simulink model "Michaels_CVModel_fast8"  (R2020a)
settings: Solver=ode23  StartTime=0.0  StopTime=30  RelTol=1e-2  EnableMultiTasking=on
model workspace (MAT data in the model file):
  Eao = 1.88
  Eesla = 0.58
  Eeslvf = 5.2
  Eesra = 0.63
  Eesrvf = 1.75
  Emaxspt = 48.75
  Epa = 0.15
  Epu = 0.04
  Esa = 0.37
  Esv = 0.013
  Evc = 0.03
  GpLV = 0
  GpRR = 11
  GpRV = 0
  GpRsa = 0
  GpV0 = 0
  GsLV = 0.007
  GsRR = 11
  GsRV = 0.022
  GsRsa = -0.05
  GsV0 = 31
  Ka = 4.4
  Lao = 0.0022
  Lav = 0.000354
  Lmt = 7.697e-05
  Lpa = 7.697e-05
  Lpv = 0.0001043
  Ltc = 8.009e-05
  P0la = 0.5
  P0lvf = 0.98
  P0pcd = 0.5
  P0ra = 0.5
  P0rvf = 0.91
  P0spt = 0.46
  PV : AO (value not decoded)
  PVao = [327.9; 100.9]
  Rao = 0.28
  Rav = 0.02
  Rla2pu = 0.5
  Rmt = 0.01
  Rpa = 0.12
  Rpa_Vals = 0.12
  Rpu = 0.006
  Rpv = 0.02
  Rra = 0.012
  Rsa = 0.74
  Rsv = 0.12
  Rtc = 0.01
  Tc = 1
  Tsys0 = 0.6
  V0la = 30
  V0lvf = 45
  V0pcd = 200
  V0ra = 25
  V0rvf = 50
  V0spt = 10
  Vdla = 15
  Vdlvf = 16
  Vdra = 15
  Vdrvf = 40
  Vdspt = 10
  Vlv0 = 100
  Vperi = 51
  Vrv0 = 105
  Vuao = 260.8
  Vupa = 91
  Vupu = 132
  Vusa = 287.4
  Vusv = 1976.1
  Vuvc = 136.17
  amin = -2
  artBrLVcontConti = []
  artBrLVcontDigi = [0 0 0 0 0 0 0 0 0 0 0 0 ... (240 elements, 1x240)]
  artBrRRConti = []
  artBrRRDigi = [0 0 0 0 0 0 0 0 0 0 1.57142857143 3.14285714286 ... (240 elements, 1x240)]
  artBrRVcontConti = []
  artBrRVcontDigi = [0 0 0 0 0 0 0 0 0 0 0 0 ... (240 elements, 1x240)]
  artBrRsaConti = []
  artBrRsaDigi = [0 0 0 0 0 0 0 0 0 0 0 0 ... (480 elements, 1x480)]
  artBrV0Conti = []
  artBrV0Digi = [0 0 0 0 0 0 0 0 0 0 0 0 ... (640 elements, 1x640)]
  atriumA = 1
  baroSampFreq = 16
  cP0la = 0.5
  cP0lvf = 0.98
  cP0ra = 0.5
  cP0rvf = 0.91
  cT = 1
  cVtotal = 5400
  clambdala = 0.13
  clambdalvf = 0.028
  clambdara = 0.13
  clambdarvf = 0.028
  deac = 0.0004
  ksys = 0.075
  lambdala = 0.065
  lambdalvf = 0.042
  lambdapcd = 0.005
  lambdara = 0.065
  lambdarvf = 0.028
  lambdaspt = 0.4
  pThor = 0
  params : object (value not decoded)
  sampleTime = 0.005
  svcPressureChange_MCS = 0
  svrMult = 1
  tStepOn = 1000000000
  t_baroOn = 1000000
  t_testBed_start = 1000000
  venk1 = 0.5
  venk2 = 0.5
symbols that are objects in the model workspace (value not decoded): PV
undefined symbols (not defined in the file): dfilt
libraries: simulink x85, fl_lib x39, nesl_utility x24, cstblocks x9, dspstat3 x9, dspobslib x5, SimscapeFluids_lib x5, sh_lib x1
(part 3 of 5)

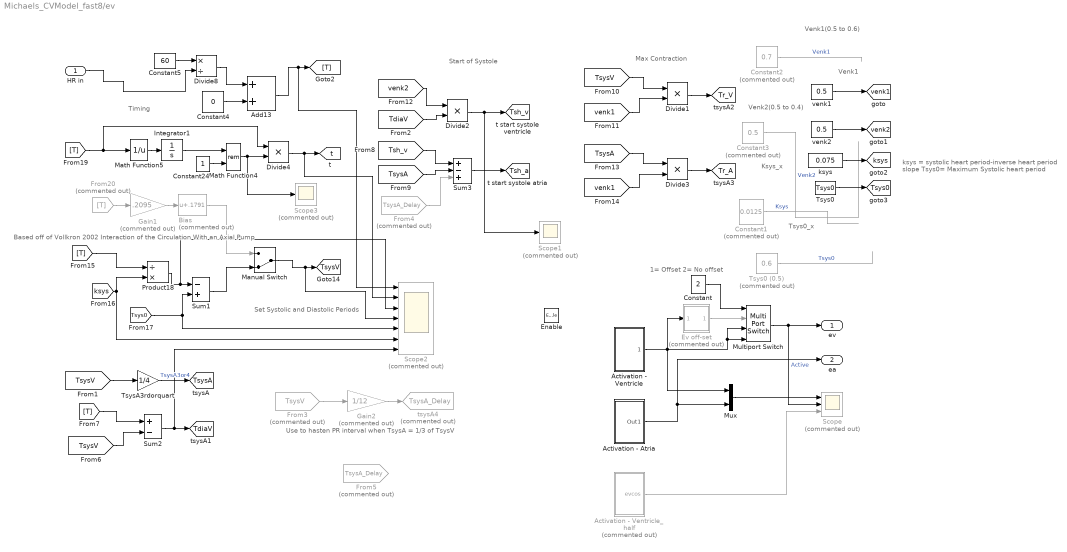
== system Michaels_CVModel_fast8/ev ==
  note: 1= Offset
      | 2= No offset
  note: ksys = systolic heart period-inverse heart period slope
      |
      | Tsys0= Maximum Systolic heart period
  note: Venk1(0.5 to 0.6)
  note: Ksys_x
  note: Timing
  note: Set Systolic and Diastolic Periods
  note: Start of Systole
  note: Max Contraction
  note: Venk1
  note: Based off of Vollkron 2002 Interaction of the Circulation With an Axial Pump
  note: Tsys0_x
  note: Venk2(0.5 to 0.4)
  note: Use to hasten PR interval when TsysA = 1/3 of TsysV
  HR in : Inport
  Enable : EnablePort
  Activation - Atria : Subsystem
  Activation - Ventricle : Subsystem
  Activation - Ventricle_half : Subsystem  Commented=on
  Add13 : Sum
  Bias : Bias  Commented=on  Bias=.1791
  Constant : Constant  Value=2
  Constant1 : Constant  Description=SettingsEV  Commented=on  Value=0.0125
  Constant2 : Constant  Description=SettingsEV  Commented=on  Value=0.7
  Constant24 : Constant
  Constant3 : Constant  Description=SettingsEV  Commented=on  Value=0.5
  Constant4 : Constant  Value=0
  Constant5 : Constant  Value=60
  Divide{1..4} (4 alike) : Product  Inputs=**
  Divide8 : Product  Inputs=*/
  Ev off-set : Subsystem  Commented=on
  From20 : From  Commented=on  GotoTag=T
      settings: CloseFcn=tagdialog Close
  From3 : From  Commented=on  GotoTag=TsysV  TagVisibility=global
      settings: CloseFcn=tagdialog Close
  From4 : From  Commented=on  GotoTag=TsysA_Delay
      settings: CloseFcn=tagdialog Close
  From5 : From  Commented=on  GotoTag=TsysA_Delay  TagVisibility=global
      settings: CloseFcn=tagdialog Close
  Gain1 : Gain  Commented=on  Gain=.2095
  Gain2 : Gain  Commented=on  Gain=1/12
  Integrator1 : Integrator
  Manual Switch : ManualSwitch  CurrentSetting=0
  Math Function4 : Math  Operator=rem  SignedPower=on  SaturateOnIntegerOverflow=on
  Math Function5 : Math  Operator=reciprocal  SignedPower=on  SaturateOnIntegerOverflow=on
  Multiport Switch : MultiPortSwitch
  Mux : Mux  Inputs=2
  Product18 : Product  Inputs=/*  InputSameDT=on  RndMeth=Zero  SaturateOnIntegerOverflow=on  OutDataTypeStr=Inherit: Same as first input
  Scope : Scope  Commented=on  NumInputPorts=3
  Scope1 : Scope  Commented=on
  Scope2 : Scope  Commented=on  NumInputPorts=7
  Scope3 : Scope  Commented=on
  Sum1 : Sum  Inputs=-+  InputSameDT=on  SaturateOnIntegerOverflow=on  OutDataTypeStr=Inherit: Same as first input
  Sum2 : Sum  Inputs=+-  InputSameDT=on  SaturateOnIntegerOverflow=on  OutDataTypeStr=Inherit: Same as first input
  Sum3 : Sum  Inputs=+-+  InputSameDT=on  SaturateOnIntegerOverflow=on  OutDataTypeStr=Inherit: Same as first input
  Tsys0 : Constant  Value=Tsys0
  Tsys0 (0.5) : Constant  Description=SettingsEV  Commented=on  Value=0.6
  TsysA3rdorquart : Gain  Gain=1/4
  ksys : Constant  Value=0.075
  tsysA4 : Goto  Commented=on  GotoTag=TsysA_Delay  TagVisibility=global
  venk1 : Constant  Value=0.5
  venk2 : Constant  Value=0.5
  ev : Outport  InitialOutput=0
  ea : Outport  Port=2  InitialOutput=0
  tag scope: TdiaV=global, Tr_A=global, Tr_V=global, Tsh_a=global, Tsh_v=global, Tsys0=global, TsysA=global, TsysV=global, ksys=global, t=global, venk1=global, venk2=global
  wires:
  [Tsys0] -> Sum1/2, Scope2/5
  Product18/1 -> Scope2/3, Sum1/1
  [ksys] -> Product18/2, Scope2/6
  Constant24/1 -> Math Function4/2
  Math Function5/1 -> Integrator1/1
  Integrator1/1 -> Math Function4/1
  [T] -> Math Function5/1, Divide4/1
  Math Function4/1 -> Scope3/1, Divide4/2
  Constant5/1 -> Divide8/1
  [TsysV] -> TsysA3rdorquart/1
  TsysA3rdorquart/1 -> [TsysA]  "TsysA3or4"
  [T] -> Sum2/1
  [TsysV] -> Sum2/2
  Sum2/1 -> Scope2/7, [TdiaV]
  [TdiaV] -> Divide2/2
  Divide2/1 -> [Tsh_v], Scope1/1
  [Tsh_v] -> Sum3/1
  [TsysA] -> Sum3/2
  Sum3/1 -> [Tsh_a]
  [TsysV] -> Divide1/1
  [venk1] -> Divide1/2
  [venk2] -> Divide2/1
  Divide1/1 -> [Tr_V]
  [TsysA] -> Divide3/1
  [venk1] -> Divide3/2
  Divide3/1 -> [Tr_A]
  [T] -> Product18/1
  Divide4/1 -> Scope2/2, [t]
  Sum1/1 -> Manual Switch/2
  Manual Switch/1 -> Scope2/4, [TsysV]
  From20/1 -> Gain1/1
  Gain1/1 -> Bias/1
  Bias/1 -> Manual Switch/1
  Mux/1 -> Scope/1
  Activation - Atria/1(Out1) -> ea/1, Mux/2
  HR in/1 -> Divide8/2
  Divide8/1 -> Add13/1
  Add13/1 -> Scope2/1, [T]
  Constant1/1 -> ?  "Ksys"
  Tsys0 (0.5)/1 -> ?  "Tsys0"
  Constant2/1 -> ?  "Venk1"
  Constant3/1 -> ?  "Venk2"
  Activation - Ventricle/1(1) -> Multiport Switch/4, Multiport Switch/3, Mux/1, Ev off-set/1(Inport)
  Activation - Ventricle_half/1(evcos) -> Scope/3
  Constant/1 -> Multiport Switch/1
  Ev off-set/1(" ") -> Multiport Switch/2
  Multiport Switch/1 -> Scope/2, ev/1  "Active"
  Constant4/1 -> Add13/2
  Gain2/1 -> tsysA4/1
  From3/1 -> Gain2/1
  From4/1 -> Sum3/3
  venk1/1 -> [venk1]
  venk2/1 -> [venk2]
  ksys/1 -> [ksys]
  Tsys0/1 -> [Tsys0]

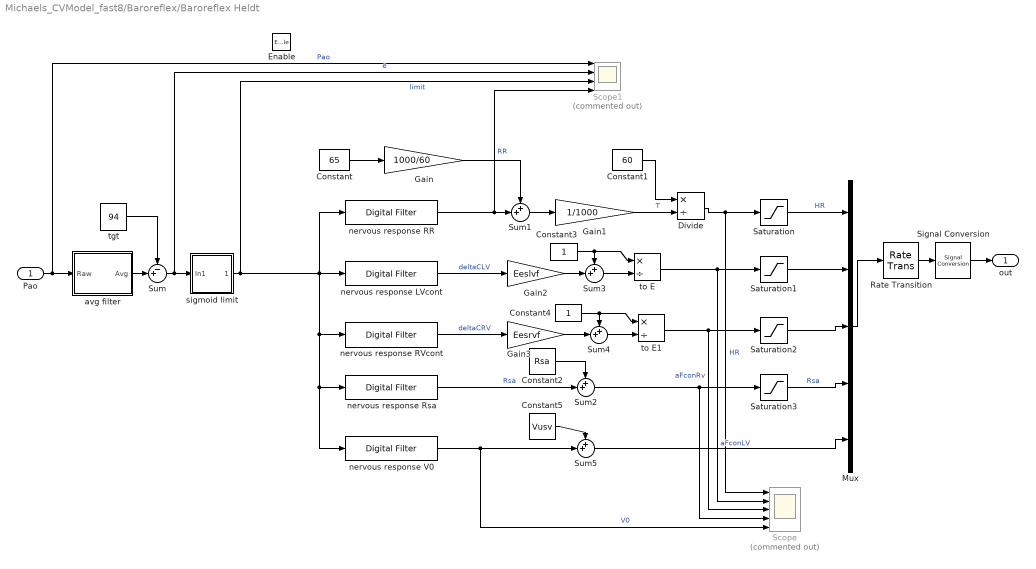
== system Michaels_CVModel_fast8/Baroreflex/Baroreflex Heldt ==
  Pao : Inport
  Enable : EnablePort
  Constant : Constant  Value=65
  Constant1 : Constant  Value=60
  Constant2 : Constant  Value=Rsa
  Constant3 : Constant
  Constant4 : Constant
  Constant5 : Constant  Value=Vusv
  Divide : Product  Inputs=*/
  Gain : Gain  Gain=1000/60
  Gain1 : Gain  Gain=1/1000
  Gain2 : Gain  Gain=Eeslvf
  Gain3 : Gain  Gain=Eesrvf
  Mux : Mux  Inputs=5
  Rate Transition : RateTransition  InitialCondition=[60,1,1,0.74,2000]
  Saturation : Saturate  UpperLimit=200  LowerLimit=30
  Saturation1 : Saturate  UpperLimit=10  LowerLimit=0.01
  Saturation2 : Saturate  UpperLimit=10  LowerLimit=0.01
  Saturation3 : Saturate  UpperLimit=inf  LowerLimit=0.001
  Scope : Scope  Commented=on  NumInputPorts=5
  Scope1 : Scope  Commented=on  NumInputPorts=4
  Signal Conversion : SignalConversion  OverrideOpt=off
  Sum : Sum  Inputs=-+|
  Sum{1..5} (5 alike) : Sum  Inputs=++|
  avg filter : Subsystem
  nervous response LVcont : dspobslib/Digital Filter  TypePopup=FIR (all zeros)  IIRFiltStruct=Direct form I  AllPoleFiltStruct=Direct form  FIRFiltStruct=Direct form  CoeffSource=Specify via dialog  NumCoeffs=artBrLVcontDigi  DenCoeffs=[1]  BiQuadCoeffs=[1 0.3 0.4 1 0.1 0.2]  LatticeCoeffs=[0.2 0.4]  denIgnore=on  FiltPerSampPopup=One filter per frame  IC=0  ICnum=0  ICden=0  roundingMode=Floor  overflowMode=off  ScaleValues=1  scaleValueFracLength=14  stageInFracLength=15  stageOutFracLength=15  FilterSource=Specify via dialog  dfiltObjectName=dfilt.dffir([1 2 1])
      settings: SourceProductBaseCode=DS
  nervous response RR : dspobslib/Digital Filter  TypePopup=FIR (all zeros)  IIRFiltStruct=Direct form I  AllPoleFiltStruct=Direct form  FIRFiltStruct=Direct form  CoeffSource=Specify via dialog  NumCoeffs=artBrRRDigi  DenCoeffs=[1]  BiQuadCoeffs=[1 0.3 0.4 1 0.1 0.2]  LatticeCoeffs=[0.2 0.4]  denIgnore=on  FiltPerSampPopup=One filter per frame  IC=0  ICnum=0  ICden=0  roundingMode=Floor  overflowMode=off  ScaleValues=1  scaleValueFracLength=14  stageInFracLength=15  stageOutFracLength=15  FilterSource=Specify via dialog  dfiltObjectName=dfilt.dffir([1 2 1])  InputProcessing=Columns as channels (frame based)
      settings: SourceProductBaseCode=DS
  nervous response RVcont : dspobslib/Digital Filter  TypePopup=FIR (all zeros)  IIRFiltStruct=Direct form I  AllPoleFiltStruct=Direct form  FIRFiltStruct=Direct form  CoeffSource=Specify via dialog  NumCoeffs=artBrRVcontDigi  DenCoeffs=[1]  BiQuadCoeffs=[1 0.3 0.4 1 0.1 0.2]  LatticeCoeffs=[0.2 0.4]  denIgnore=on  FiltPerSampPopup=One filter per frame  IC=0  ICnum=0  ICden=0  roundingMode=Floor  overflowMode=off  ScaleValues=1  scaleValueFracLength=14  stageInFracLength=15  stageOutFracLength=15  FilterSource=Specify via dialog  dfiltObjectName=dfilt.dffir([1 2 1])
      settings: SourceProductBaseCode=DS
  nervous response Rsa : dspobslib/Digital Filter  TypePopup=FIR (all zeros)  IIRFiltStruct=Direct form I  AllPoleFiltStruct=Direct form  FIRFiltStruct=Direct form  CoeffSource=Specify via dialog  NumCoeffs=artBrRsaDigi  DenCoeffs=[1]  BiQuadCoeffs=[1 0.3 0.4 1 0.1 0.2]  LatticeCoeffs=[0.2 0.4]  denIgnore=on  FiltPerSampPopup=One filter per frame  IC=0  ICnum=0  ICden=0  roundingMode=Floor  overflowMode=off  ScaleValues=1  scaleValueFracLength=14  stageInFracLength=15  stageOutFracLength=15  FilterSource=Specify via dialog  dfiltObjectName=dfilt.dffir([1 2 1])
      settings: SourceProductBaseCode=DS
  nervous response V0 : dspobslib/Digital Filter  TypePopup=FIR (all zeros)  IIRFiltStruct=Direct form I  AllPoleFiltStruct=Direct form  FIRFiltStruct=Direct form  CoeffSource=Specify via dialog  NumCoeffs=artBrV0Digi  DenCoeffs=[1]  BiQuadCoeffs=[1 0.3 0.4 1 0.1 0.2]  LatticeCoeffs=[0.2 0.4]  denIgnore=on  FiltPerSampPopup=One filter per frame  IC=0  ICnum=0  ICden=0  roundingMode=Floor  overflowMode=off  ScaleValues=1  scaleValueFracLength=14  stageInFracLength=15  stageOutFracLength=15  FilterSource=Specify via dialog  dfiltObjectName=dfilt.dffir([1 2 1])
      settings: SourceProductBaseCode=DS
  sigmoid limit : Subsystem
  tgt : Constant  Value=94
  to E : Product  Inputs=*/
  to E1 : Product  Inputs=*/
  out : Outport  InitialOutput=[60,1,1,0.74,2000]
  wires:
  Pao/1 -> avg filter/1(Raw), Scope1/1  "Pao"
  tgt/1 -> Sum/1
  avg filter/1(Avg) -> Sum/2
  Sum/1 -> Scope1/2, sigmoid limit/1(In1)  "e"
  nervous response RR/1 -> Sum1/2, Scope1/4  "RR"
  nervous response LVcont/1 -> Gain2/1  "deltaCLV"
  nervous response Rsa/1 -> Sum2/2  "Rsa"
  nervous response V0/1 -> Scope/5, Sum5/2  "V0"
  Constant/1 -> Gain/1
  Gain/1 -> Sum1/1
  Sum1/1 -> Gain1/1
  Divide/1 -> Saturation/1, Scope/1  "HR"
  Saturation/1 -> Mux/1  "HR"
  Constant1/1 -> Divide/1
  Gain1/1 -> Divide/2  "T"
  sigmoid limit/1(Out1) -> Scope1/3, nervous response RR/1, nervous response LVcont/1, nervous response RVcont/1, nervous response Rsa/1, nervous response V0/1  "limit"
  Constant2/1 -> Sum2/1
  Sum2/1 -> Scope/4, Saturation3/1
  Constant3/1 -> Sum3/1, to E/1
  Sum3/1 -> to E/2
  Gain2/1 -> Sum3/2
  to E/1 -> Scope/2, Saturation1/1  "aFconLV"
  Constant4/1 -> Sum4/1, to E1/1
  Sum4/1 -> to E1/2
  Gain3/1 -> Sum4/2
  nervous response RVcont/1 -> Gain3/1  "deltaCRV"
  to E1/1 -> Scope/3, Saturation2/1  "aFconRv"
  Saturation1/1 -> Mux/2
  Saturation2/1 -> Mux/3
  Saturation3/1 -> Mux/4  "Rsa"
  Mux/1 -> Rate Transition/1
  Constant5/1 -> Sum5/1
  Sum5/1 -> Mux/5
  Rate Transition/1 -> Signal Conversion/1
  Signal Conversion/1 -> out/1

== system Michaels_CVModel_fast8/Baroreflex/Baroreflex Heldt cont ==
  Pao : Inport
  Enable : EnablePort
  Constant : Constant  Value=50
  Constant1 : Constant  Value=60
  Constant2 : Constant  Value=Rsa
  Constant3 : Constant
  Constant4 : Constant
  Constant5 : Constant  Value=Vusv
  Divide : Product  Inputs=*/
  Filter : Subsystem
  Gain : Gain  Gain=1000/60
  Gain1 : Gain  Gain=1/1000
  Gain2 : Gain  Gain=Eeslvf
  Gain3 : Gain  Gain=Eesrvf
  LTI System : cstblocks/LTI System  sys=artBrRRConti  IC=[]
  LTI System1 : cstblocks/LTI System  sys=artBrLVcontConti  IC=[]
  LTI System2 : cstblocks/LTI System  sys=artBrRVcontConti  IC=[]
  LTI System3 : cstblocks/LTI System  sys=artBrRsaConti  IC=[]
  LTI System4 : cstblocks/LTI System  sys=artBrV0Conti  IC=[]
  Mux : Mux  Inputs=5
  Saturation : Saturate  UpperLimit=200  LowerLimit=30
  Saturation1 : Saturate  UpperLimit=10  LowerLimit=0.01
  Saturation2 : Saturate  UpperLimit=10  LowerLimit=0.01
  Saturation3 : Saturate  UpperLimit=inf  LowerLimit=0.001
  Saturation4 : Saturate  UpperLimit=inf  LowerLimit=0.001
  Scope : Scope  Commented=on  NumInputPorts=5
  Scope1 : Scope  Commented=on  NumInputPorts=4
  Sum : Sum  Inputs=-+|
  Sum{1..5} (5 alike) : Sum  Inputs=++|
  sigmoid limit : Subsystem
  tgt : Constant  Value=95
  to E : Product  Inputs=*/
  to E1 : Product  Inputs=*/
  out : Outport  InitialOutput=[60,1,1,0.74,2000]
  wires:
  Pao/1 -> Filter/1(Raw), Scope1/1  "Pao"
  tgt/1 -> Sum/1
  Filter/1(Filtered) -> Sum/2
  Sum/1 -> Scope1/2, sigmoid limit/1(In1)  "e"
  LTI System/1 -> Sum1/2, Scope1/4  "deltaRR"
  LTI System1/1 -> Gain2/1  "deltaCLV"
  LTI System3/1 -> Sum2/2  "deltaRsa"
  LTI System4/1 -> Scope/5, Sum5/2  "deltaV0"
  Constant/1 -> Gain/1
  Gain/1 -> Sum1/1
  Sum1/1 -> Gain1/1
  Divide/1 -> Saturation/1, Scope/1  "HR"
  Saturation/1 -> Mux/1  "HR"
  Constant1/1 -> Divide/1
  Gain1/1 -> Divide/2  "T"
  sigmoid limit/1(Out1) -> Scope1/3, LTI System3/1, LTI System4/1, LTI System2/1, LTI System/1, LTI System1/1  "limit"
  Constant2/1 -> Sum2/1
  Sum2/1 -> Scope/4, Saturation3/1
  Constant3/1 -> Sum3/1, to E/1
  Sum3/1 -> to E/2
  Gain2/1 -> Sum3/2
  to E/1 -> Scope/2, Saturation1/1  "aFconLV"
  Constant4/1 -> Sum4/1, to E1/1
  Sum4/1 -> to E1/2
  Gain3/1 -> Sum4/2
  LTI System2/1 -> Gain3/1  "deltaCRV"
  to E1/1 -> Scope/3, Saturation2/1  "aFconRv"
  Saturation1/1 -> Mux/2
  Saturation2/1 -> Mux/3
  Saturation3/1 -> Mux/4  "Rsa"
  Mux/1 -> out/1
  Constant5/1 -> Sum5/1
  Sum5/1 -> Saturation4/1
  Saturation4/1 -> Mux/5

== system Michaels_CVModel_fast8/Baroreflex/Baroreflex Lu ==
  note: Rsa Trans Fn
  note: HR Tans Fn
  note: old 1.099
  note: .8
  note: 1.1
  Pao : Inport
  Vsa : Inport  Port=2
  Enable : EnablePort
  Add : Sum
  Baroreceptor : TransferFcn  Numerator=[0.036 1]  Denominator=[0.0018^2 0.0036 1]
  Constant : Constant  Value=amin
  Constant1 : Constant  Value=Ka
  Constant3 : Constant  Value=Vusv
  Contractility Function : MATLAB Function  TreatAsAtomicUnit=on
  Fcon : MATLAB Function  TreatAsAtomicUnit=on
  Fhr : Scope  Commented=on  NumInputPorts=2
  FhrS : MATLAB Function  TreatAsAtomicUnit=on
  FhrV : MATLAB Function  TreatAsAtomicUnit=on
  Fvaso : MATLAB Function  TreatAsAtomicUnit=on
  Gain : Gain  Gain=1.05  SampleTime=0.01
  Gain1 : Gain  Gain=0.8
  Gain2 : Gain  Gain=0.95
  Gain3 : Gain  Gain=1.0
  Gain4 : Gain  Gain=1.1
  HR Offset : Constant  Value=-40
  HR transfer Function : MATLAB Function  TreatAsAtomicUnit=on
  Mux : Mux  Inputs=5
  Rsa Trans Fn : MATLAB Function  TreatAsAtomicUnit=on
  Saturation : Saturate  UpperLimit=inf  LowerLimit=0
  Scope : Scope  Commented=on
  Transfer Fn Ncon : cstblocks/LTI System  sys=tf(1,[10 1],'inputdelay',3);  IC=[]
  Transfer Fn NrS : cstblocks/LTI System  sys=tf(1,[10 1],'inputdelay',3);  IC=[]
  Transfer Fn Nrv : cstblocks/LTI System  sys=tf(1,[1.8 1],'inputdelay',0.2);  IC=[]
  Transfer Fn NvasoS : cstblocks/LTI System  sys=tf(1,[6 1],'inputdelay',3);  IC=[]
  out : Outport  InitialOutput=[60,1,1,0.74,2000]
  wires:
  Mux/1 -> out/1
  Pao/1 -> Gain/1
  Gain/1 -> Baroreceptor/1
  Baroreceptor/1 -> Gain3/1, Gain1/1, Gain2/1, Gain4/1
  Gain1/1 -> Transfer Fn Nrv/1
  Gain3/1 -> Transfer Fn NrS/1
  Gain2/1 -> Transfer Fn NvasoS/1
  Transfer Fn Nrv/1 -> FhrV/1(Nhrv)
  Transfer Fn NrS/1 -> FhrS/1(Nhrs)
  Transfer Fn NvasoS/1 -> Fvaso/1(Nvaso)
  FhrV/1(Fhrv) -> HR transfer Function/1(Fhrv), Fhr/1  "FHrv"
  FhrS/1(Fhrs) -> HR transfer Function/2(Fhrs), Fhr/2  "FHrs"
  Fvaso/1(Fvaso) -> Rsa Trans Fn/1(Fvaso)
  Rsa Trans Fn/1(Rsa) -> Mux/4
  Vsa/1 -> Rsa Trans Fn/2(Vsa)
  Gain4/1 -> Transfer Fn Ncon/1
  Transfer Fn Ncon/1 -> Fcon/1(Nvaso)
  Fcon/1(Fvaso) -> Contractility Function/1(Fcon), Scope/1
  Contractility Function/1(aFcon) -> Saturation/1
  Constant/1 -> Contractility Function/2(amin)
  Saturation/1 -> Mux/2, Mux/3
  Constant1/1 -> Contractility Function/3(Ka)
  HR transfer Function/1(HR) -> Add/1
  Add/1 -> Mux/1
  HR Offset/1 -> Add/2
  Constant3/1 -> Mux/5

== system Michaels_CVModel_fast8/Baroreflex/No Baroreflex ==
  note: Default = 1976.1
  note: Notes;
      |
      | Defaults Values:
      | Rsa = 0.74
      | Vusv= 1976.1
      |
      | For SBP120 at 30secs;
      | Normal Valves:
      | Rsa = 0.665
      | Vusv= 2000
      |
      | AS1cm;
      | Rsa = 0.66
      | Vusv= 1850
      |
      | AS1cm_MR0.2;
      | Rsa = 0.75
      | Vusv= 1650
      |
      | AS1cm_MR0.5 (@36secs);
      | Rsa = 0.905
      | Vusv= 1000
      | Vlv IC 160mls,Vla IC 80mls
      |
      | Eao switch on.
  note: Default = 0.74
  Enable : EnablePort
  Constant1 : Constant
  Constant2 : Constant  Description=Settings1  Value=0.74
  Constant3 : Constant  Description=Settings1  Value=1976.1
  Constant5 : Constant  Value=70
  Constant8 : Constant  Value=cT
  Divide8 : Product  Inputs=*/
  Mux : Mux  Inputs=5
  out : Outport  InitialOutput=[60,1,1,0.74,2000]
  wires:
  Constant8/1 -> Divide8/2
  Constant5/1 -> Divide8/1
  Mux/1 -> out/1
  Divide8/1 -> Mux/1  "HR"
  Constant1/1 -> Mux/2, Mux/3  "aFcon"
  Constant2/1 -> Mux/4  "Rsa"
  Constant3/1 -> Mux/5  "Vusv"

== system Michaels_CVModel_fast8/Graphs and Scopes/LA PV Loop Delay_MS ==
  X : Inport
  Y : Inport  Port=2
  Enable : EnablePort
  LA PV Delay_MS : simulink/Sinks/XY Graph  xmin=20  xmax=100  ymin=0  ymax=40  st=0.01
  wires:
  X/1 -> LA PV Delay_MS/1
  Y/1 -> LA PV Delay_MS/2

== system Michaels_CVModel_fast8/Graphs and Scopes/LA PV Loop Delay_MS1 ==
  X : Inport
  Y : Inport  Port=2
  Enable : EnablePort
  LA PV Delay_MS : simulink/Sinks/XY Graph  xmin=20  xmax=100  ymin=0  ymax=40  st=0.01
  wires:
  Y/1 -> LA PV Delay_MS/2
  X/1 -> LA PV Delay_MS/1

== system Michaels_CVModel_fast8/Graphs and Scopes/LA PV Loop_MS ==
  X : Inport
  Y : Inport  Port=2
  Enable : EnablePort
  LA PV Loop_MS : simulink/Sinks/XY Graph  xmin=0  xmax=100  ymin=0  ymax=40  st=0.005
  wires:
  X/1 -> LA PV Loop_MS/1
  Y/1 -> LA PV Loop_MS/2

== system Michaels_CVModel_fast8/Graphs and Scopes/LV PV Loop _Delay ==
  X : Inport
  Y : Inport  Port=2
  Enable : EnablePort
  Add : Sum  Commented=on  Inputs=+-
  Divide : Product  Commented=on  Inputs=*/
  LV PV Loop Delay_MS : simulink/Sinks/XY Graph  xmin=-10  xmax=200  ymin=-10  ymax=200  st=0.01
  MinMax : MinMax  Commented=on  Function=max
  MinMax1 : MinMax  Commented=on
  Scope : Scope  Commented=on  NumInputPorts=2
  Scope1 : Scope  Commented=on  NumInputPorts=2
  wires:
  X/1 -> MinMax1/1, MinMax/1, LV PV Loop Delay_MS/1
  Y/1 -> LV PV Loop Delay_MS/2
  MinMax1/1 -> Add/2, Scope/1
  MinMax/1 -> Divide/2, Add/1, Scope/2
  Add/1 -> Divide/1
  Divide/1 -> Scope1/1

== system Michaels_CVModel_fast8/Graphs and Scopes/LV PV Loop _Delay1 ==
  X : Inport
  Y : Inport  Port=2
  Enable : EnablePort
  Add : Sum  Commented=on  Inputs=+-
  Divide : Product  Commented=on  Inputs=*/
  LV PV Loop Delay_MS : simulink/Sinks/XY Graph  xmin=-10  xmax=200  ymin=-10  ymax=200  st=0.01
  MinMax : MinMax  Commented=on  Function=max
  MinMax1 : MinMax  Commented=on
  Scope : Scope  Commented=on  NumInputPorts=2
  Scope1 : Scope  Commented=on  NumInputPorts=2
  wires:
  Divide/1 -> Scope1/1
  Add/1 -> Divide/1
  MinMax/1 -> Scope/2, Add/1, Divide/2
  MinMax1/1 -> Scope/1, Add/2
  Y/1 -> LV PV Loop Delay_MS/2
  X/1 -> LV PV Loop Delay_MS/1, MinMax/1, MinMax1/1

== system Michaels_CVModel_fast8/Graphs and Scopes/LV PV Loop _Delay2 ==
  X : Inport
  Y : Inport  Port=2
  Enable : EnablePort
  Add : Sum  Commented=on  Inputs=+-
  Divide : Product  Commented=on  Inputs=*/
  LV PV Loop Delay_MS : simulink/Sinks/XY Graph  xmin=-10  xmax=200  ymin=-10  ymax=200  st=0.002
  MinMax : MinMax  Commented=on  Function=max
  MinMax1 : MinMax  Commented=on
  Scope : Scope  Commented=on  NumInputPorts=2
  Scope1 : Scope  Commented=on  NumInputPorts=2
  wires:
  X/1 -> MinMax1/1, MinMax/1, LV PV Loop Delay_MS/1
  Y/1 -> LV PV Loop Delay_MS/2
  MinMax1/1 -> Add/2, Scope/1
  MinMax/1 -> Divide/2, Add/1, Scope/2
  Add/1 -> Divide/1
  Divide/1 -> Scope1/1

== system Michaels_CVModel_fast8/Graphs and Scopes/LV PV Loop_MS ==
  X : Inport
  Y : Inport  Port=2
  Enable : EnablePort
  LV PV Loop_MS : simulink/Sinks/XY Graph  xmin=-10  xmax=200  ymin=-10  ymax=250  st=0.01
  wires:
  X/1 -> LV PV Loop_MS/1
  Y/1 -> LV PV Loop_MS/2

== system Michaels_CVModel_fast8/Graphs and Scopes/LVEDP ==
  X : Inport
  Enable : EnablePort
  Outport : Outport  SampleTime=0.001
  wires:
  X/1 -> Outport/1

== system Michaels_CVModel_fast8/Graphs and Scopes/MPGX ==
  X : Inport
  Enable : EnablePort  StatesWhenEnabling=reset
  Outport : Outport
  wires:
  X/1 -> Outport/1

== system Michaels_CVModel_fast8/Graphs and Scopes/MPGX1 ==
  X : Inport
  Enable : EnablePort  StatesWhenEnabling=reset
  Outport : Outport
  wires:
  X/1 -> Outport/1

== system Michaels_CVModel_fast8/Graphs and Scopes/RA PV Loop ==
  X : Inport
  Y : Inport  Port=2
  Enable : EnablePort
  RA PV Loop_MS : simulink/Sinks/XY Graph  xmin=10  xmax=100  ymin=0  ymax=30  st=0.01
  wires:
  X/1 -> RA PV Loop_MS/1
  Y/1 -> RA PV Loop_MS/2

== system Michaels_CVModel_fast8/Graphs and Scopes/RV PV Loop Delay_MS ==
  X : Inport
  Y : Inport  Port=2
  Enable : EnablePort
  RV PV Loop Delay_MS : simulink/Sinks/XY Graph  xmin=-10  xmax=150  ymin=-10  ymax=60  st=0.01
  wires:
  Y/1 -> RV PV Loop Delay_MS/2
  X/1 -> RV PV Loop Delay_MS/1

== system Michaels_CVModel_fast8/Graphs and Scopes/RV PV Loop_MS ==
  X : Inport
  Y : Inport  Port=2
  Enable : EnablePort
  RV PV Loop_MS : simulink/Sinks/XY Graph  xmin=-10  xmax=150  ymin=-10  ymax=60  st=0.01
  wires:
  X/1 -> RV PV Loop_MS/1
  Y/1 -> RV PV Loop_MS/2

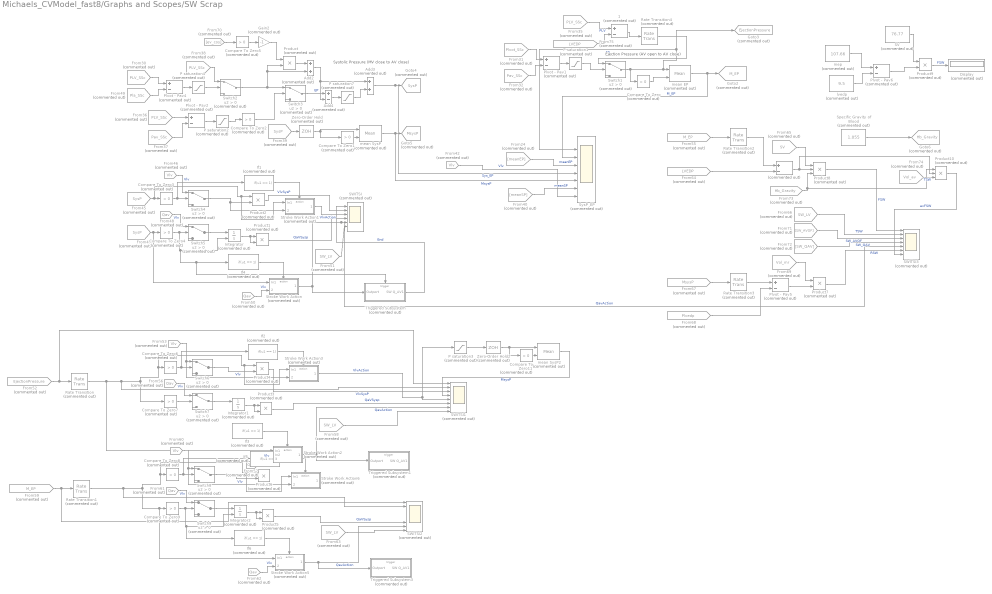
== system Michaels_CVModel_fast8/Graphs and Scopes/SW Scrap ==
  note: Ejection Pressure (AV open to AV close)
  note: Systolic Pressure (MV close to AV close)
  " " : Sum  Commented=on  Inputs=+-
  " 1" : Sum  Commented=on  Inputs=+-
  Add2 : Sum  Commented=on
  Add3 : Sum  Commented=on
  Add4 : Sum  Commented=on  Inputs=+-
  Compare To Zero{,1..9,11} (11 alike) : simulink/Logic and Bit Operations/Compare To Zero  Commented=on  relop=>  OutDataTypeStr=boolean
  Display : Display  Commented=on
  From24 : From  Commented=on  GotoTag=meanEP  TagVisibility=global
  From{30,35..36,38} (4 alike) : From  Commented=on  GotoTag=PLV_SSc  TagVisibility=global
      From35 settings: CloseFcn=tagdialog Close
      From38 settings: CloseFcn=tagdialog Close
  From31 : From  Commented=on  GotoTag=Plvot_SSc  TagVisibility=global
  From32 : From  Commented=on  GotoTag=Pav_SSc  TagVisibility=global
  From37 : From  Commented=on  GotoTag=Pav_SSc  TagVisibility=global
  From39 : From  Commented=on  GotoTag=SysP  TagVisibility=global
  From40 : From  Commented=on  GotoTag=meanSP  TagVisibility=global
  From{42,46,53,60} (4 alike) : From  Commented=on  GotoTag=Vlv  TagVisibility=global
      settings: CloseFcn=tagdialog Close
  From45 : From  Commented=on  GotoTag=SysP  TagVisibility=global
  From47 : From  Commented=on  GotoTag=SysP  TagVisibility=global
  From{48,50,56..57,61..62} (6 alike) : From  Commented=on  GotoTag=Qav  TagVisibility=global
      settings: CloseFcn=tagdialog Close
  From49 : From  Commented=on  GotoTag=Pla_SSc  TagVisibility=global
      settings: CloseFcn=tagdialog Close
  From{51,58,63,66} (4 alike) : From  Commented=on  GotoTag=SW_LV  TagVisibility=global
  From52 : From  Commented=on  GotoTag=EjectionPressure  TagVisibility=global
  From55 : From  Commented=on  GotoTag=M_EP  TagVisibility=global
  From59 : From  Commented=on  GotoTag=M_EP  TagVisibility=global
  From64 : From  Commented=on  GotoTag=LVEDP  TagVisibility=global
  From65 : From  Commented=on  GotoTag=SV  TagVisibility=global
  From67 : From  Commented=on  GotoTag=MsysP
  From68 : From  Commented=on  GotoTag=Plvedp  TagVisibility=global
  From69 : From  Commented=on  GotoTag=Vol_mr  TagVisibility=global
  From70 : From  Commented=on  GotoTag=ev_cos  TagVisibility=global
  From71 : From  Commented=on  GotoTag=SW_AVOF  TagVisibility=global
  From72 : From  Commented=on  GotoTag=SW_QAV
  From73 : From  Commented=on  GotoTag=Hb_Gravity  TagVisibility=global
  From74 : From  Commented=on  GotoTag=Vol_av  TagVisibility=global
  From75 : From  Commented=on  GotoTag=LVEDP  TagVisibility=global
  Gain2 : Gain  Commented=on  Gain=-1
  Goto2 : Goto  Commented=on  GotoTag=M_EP  TagVisibility=global
  Goto3 : Goto  Commented=on  GotoTag=EjectionPressure  TagVisibility=global
  Goto4 : Goto  Commented=on  GotoTag=SysP  TagVisibility=global
  Goto5 : Goto  Commented=on  GotoTag=MsysP  TagVisibility=global
  Goto6 : Goto  Commented=on  GotoTag=Hb_Gravity  TagVisibility=global
  If{1..6} (6 alike) : If  Commented=on  IfExpression=u1 == 1  ShowElse=off
  Integrator : Integrator  Commented=on  ExternalReset=rising
  Integrator1 : Integrator  Commented=on  ExternalReset=either
  Integrator2 : Integrator  Commented=on  ExternalReset=rising
  P saturation{1,3..4,7} (4 alike) : Saturate  Commented=on  UpperLimit=inf  LowerLimit=0
  P saturation2 : Saturate  Commented=on  UpperLimit=inf  LowerLimit=-0.2
  Plvot - Pav{1..2,4..6} (5 alike) : Sum  Commented=on  Inputs=+-
  Product{,1..7,9} (9 alike) : Product  Commented=on
  Product10 : Product  Commented=on  Inputs=3
  Product8 : Product  Commented=on  Inputs=3
  Rate Transition{,1..4} (5 alike) : RateTransition  Commented=on
  SV : Constant  Commented=on  Value=76.77
  SWITSI : Scope  Commented=on  NumInputPorts=6
  SWITSI1 : Scope  Commented=on  NumInputPorts=8
  SWITSI2 : Scope  Commented=on  NumInputPorts=8
  SWITSI3 : Scope  Commented=on  NumInputPorts=8
  Specific Gravity of Blood : Constant  Commented=on  Value=1.055
  Stroke Work Action : Subsystem  Commented=on  TreatAsAtomicUnit=on
  Stroke Work Action1 : Subsystem  Commented=on  TreatAsAtomicUnit=on
  Stroke Work Action2 : Subsystem  Commented=on  TreatAsAtomicUnit=on
  Stroke Work Action3 : Subsystem  Commented=on  TreatAsAtomicUnit=on
  Stroke Work Action5 : Subsystem  Commented=on  TreatAsAtomicUnit=on
  Stroke Work Action6 : Subsystem  Commented=on  TreatAsAtomicUnit=on
  Switch{1..9} (9 alike) : Switch  Commented=on  Criteria=u2 > Threshold
  SysP_EP : Scope  Commented=on  NumInputPorts=8
  Triggered Subsystem : Subsystem  Commented=on  TreatAsAtomicUnit=on
  Triggered Subsystem1 : Subsystem  Commented=on  TreatAsAtomicUnit=on
  Triggered Subsystem3 : Subsystem  Commented=on  TreatAsAtomicUnit=on
  Zero-Order Hold : ZeroOrderHold  Commented=on  SampleTime=0.0001
  Zero-Order Hold2 : ZeroOrderHold  Commented=on  SampleTime=0.0001
  lvedp : Constant  Commented=on  Value=9.5
  mean EP : dspstat3/Mean  Commented=on  run=on  reset_popup=Either edge  directionMode=Each column  dimension=1  roiEnable=off  roiType=Rectangles  roiPortion=Entire ROI  roiOutput=Individual statistics for each ROI  roiFlag=off  roundingMode=Floor  overflowMode=off  outputDataTypeStr=Inherit: Same as accumulator  outputMin=[]  outputMax=[]  outputLastDataTypeStr=Inherit: Same as accumulator
  mean SysP : dspstat3/Mean  Commented=on  run=on  reset_popup=Either edge  directionMode=Each column  dimension=1  roiEnable=off  roiType=Rectangles  roiPortion=Entire ROI  roiOutput=Individual statistics for each ROI  roiFlag=off  roundingMode=Floor  overflowMode=off  outputDataTypeStr=Inherit: Same as accumulator  outputMin=[]  outputMax=[]  outputLastDataTypeStr=Inherit: Same as accumulator
  mean SysP2 : dspstat3/Mean  Commented=on  run=on  reset_popup=Either edge  directionMode=Each column  dimension=1  roiEnable=off  roiType=Rectangles  roiPortion=Entire ROI  roiOutput=Individual statistics for each ROI  roiFlag=off  roundingMode=Floor  overflowMode=off  outputDataTypeStr=Inherit: Same as accumulator  outputMin=[]  outputMax=[]  outputLastDataTypeStr=Inherit: Same as accumulator
  mep : Constant  Commented=on  Value=107.66
  wires:
  Gain2/1 -> Product/1
  From39/1 -> Zero-Order Hold/1
  From52/1 -> SWITSI1/1, Rate Transition/1
  lvedp/1 -> Plvot - Pav6/2
  From57/1 -> Stroke Work Action2/3(Inport2)  "Vlv"
  Switch3/1 -> Add4/1  "EP"
  Product10/1 -> SWITSI3/7  "avFSW"
  Switch1/1 -> SysP_EP/2, Goto3/1, mean EP/1, Compare To Zero/1  "EP"
  From32/1 -> Plvot - Pav1/2
  From56/1 -> Switch7/1  "Vlv"
  Product5/1 -> SWITSI2/6  "QaVSysp"
  Rate Transition/1 -> Stroke Work Action2/1(In1), SWITSI1/2, Product4/1, Stroke Work Action3/1(In1), Compare To Zero6/1, Compare To Zero7/1
  From50/1 -> Stroke Work Action/2(Inport2)  "Vlv"
  Specific Gravity of Blood/1 -> Goto6/1
  Product8/1 -> SWITSI3/1  "FSW"
  Compare To Zero2/1 -> Switch3/2
  Zero-Order Hold2/1 -> mean SysP2/1, Compare To Zero11/1
  From73/1 -> Product10/1, Product8/3
  From64/1 -> " "/2
  P saturation3/1 -> Zero-Order Hold2/1
  From42/1 -> SysP_EP/8  "Vlv"
  Add4/1 -> P saturation7/1
  From74/1 -> Product10/3  "TSW"
  If5/1 -> Stroke Work Action6/Action
  From40/1 -> SysP_EP/7  "meanSP"
  Compare To Zero3/1 -> Switch4/2, If1/1
  " "/1 -> Product10/2, Product8/2
  Rate Transition1/1 -> Stroke Work Action5/1(In1), Compare To Zero9/1, Compare To Zero8/1, Stroke Work Action6/1(In1), Product6/1, SWITSI2/2
  Stroke Work Action5/1(Outport) -> Triggered Subsystem3/1(Outport), SWITSI2/7  "QavAction"
  Integrator/1 -> Product1/2, Product1/1
  Switch2/1 -> Switch3/1, Product/2, Add2/2
  Product7/1 -> SWITSI3/6  "RSW"
  Rate Transition3/1 -> Plvot - Pav5/1
  From67/1 -> Rate Transition3/1
  Compare To Zero7/1 -> Switch7/2
  From46/1 -> Switch4/1  "Vlv"
  Switch9/1 -> Integrator2/1
  P saturation7/1 -> Add3/2
  Compare To Zero1/1 -> mean SysP/2
  From66/1 -> SWITSI3/2  "TSW"
  From60/1 -> Stroke Work Action6/2(Inport2), Switch8/1  "Vlv"
  P saturation1/1 -> Switch1/2
  From59/1 -> Rate Transition1/1, SWITSI2/1
  Rate Transition2/1 -> " "/1
  From65/1 -> Product8/1
  Compare To Zero5/1 -> Gain2/1
  Plvot - Pav5/1 -> Product7/2
  Compare To Zero8/1 -> Switch8/2, If5/1
  From70/1 -> Compare To Zero5/1
  Triggered Subsystem/1(SW Q_AV1) -> SWITSI/1  "End"
  SV/1 -> Product9/1
  Add3/1 -> SysP_EP/5, Goto4/1  "Sys_EP"
  Zero-Order Hold/1 -> mean SysP/1, Compare To Zero1/1
  Plvot - Pav4/1 -> P saturation4/1
  From47/1 -> Stroke Work Action/1(In1), Compare To Zero4/1
  Compare To Zero/1 -> mean EP/2
  If1/1 -> Stroke Work Action1/Action
  Switch4/1 -> Product2/2, Stroke Work Action1/2(Inport2)
  From36/1 -> Plvot - Pav2/1
  From49/1 -> Plvot - Pav4/2
  From30/1 -> Plvot - Pav4/1
  Product/1 -> Add2/1
  Compare To Zero9/1 -> If6/1, Integrator2/2, Switch9/2
  From31/1 -> Plvot - Pav1/1
  P saturation2/1 -> Compare To Zero2/1
  From24/1 -> SysP_EP/4  "meanEP"
  mean EP/1 -> SysP_EP/3, Goto2/1  "M_EP"
  mean SysP/1 -> SysP_EP/6, Goto5/1  "MsysP"
  Compare To Zero4/1 -> Triggered Subsystem/Trigger, If4/1, Integrator/2, Switch5/2
  If3/1 -> Stroke Work Action2/Action
  Compare To Zero11/1 -> mean SysP2/2
  Switch5/1 -> Integrator/1
  From48/1 -> Switch5/1  "Vlv"
  If4/1 -> Stroke Work Action/Action
  From72/1 -> SWITSI3/4  "SW_QAV"
  Plvot - Pav6/1 -> Product9/2
  P saturation4/1 -> Switch2/2
  From45/1 -> Stroke Work Action1/1(In1), Product2/1, Compare To Zero3/1
  From63/1 -> SWITSI2/8
  Switch7/1 -> Integrator1/1
  Plvot - Pav1/1 -> P saturation1/1
  From38/1 -> Switch2/1
  mep/1 -> Plvot - Pav6/1
  Switch8/1 -> Product6/2
  Compare To Zero6/1 -> If2/1, Switch6/2
  Switch6/1 -> Product4/2
  From55/1 -> Rate Transition2/1
  From37/1 -> Plvot - Pav2/2
  If6/1 -> Stroke Work Action5/Action
  Stroke Work Action2/1(Outport) -> SWITSI1/7, Triggered Subsystem1/1(Outport)  "QavAction"
  " 1"/1 -> Rate Transition4/1
  From62/1 -> Stroke Work Action5/2(Inport2)  "Vlv"
  Stroke Work Action3/1(Outport) -> SWITSI1/5, P saturation3/1  "VlvAction"
  If2/1 -> Stroke Work Action3/Action
  Integrator1/1 -> Product3/1, Product3/2
  Product4/1 -> SWITSI1/3  "VlvSysP"
  From53/1 -> Stroke Work Action3/2(Inport2), Switch6/1  "Vlv"
  From58/1 -> SWITSI1/8
  Integrator2/1 -> Product5/2, Product5/1
  From51/1 -> SWITSI/6
  From61/1 -> Switch9/1  "Vlv"
  Plvot - Pav2/1 -> P saturation2/1
  Add2/1 -> Add3/1, Add4/2
  mean SysP2/1 -> SWITSI1/4  "MsysP"
  Stroke Work Action1/1(Outport) -> SWITSI/3  "VlvAction"
  From71/1 -> SWITSI3/3  "SW_AVOF"
  Product3/1 -> SWITSI1/6  "QaVSysp"
  From68/1 -> Plvot - Pav5/2
  From69/1 -> Product7/1
  Product9/1 -> Display/1  "FSW"
  Stroke Work Action/1(Outport) -> Triggered Subsystem/1(Outport), SWITSI3/5, SWITSI/5  "QavAction"
  Product2/1 -> SWITSI/2  "VlvSysP"
  Product1/1 -> SWITSI/4  "QaVSysp"
  From35/1 -> " 1"/1  "PLV"
  From75/1 -> " 1"/2
  Rate Transition4/1 -> Switch1/1

== system Michaels_CVModel_fast8/Graphs and Scopes/mLAP ==
  X : Inport
  Enable : EnablePort
  Outport : Outport  SampleTime=0.001
  wires:
  X/1 -> Outport/1

== system Michaels_CVModel_fast8/Graphs and Scopes/mLAP1 ==
  X : Inport
  Enable : EnablePort
  Outport : Outport  SampleTime=0.001
  wires:
  X/1 -> Outport/1

== system Michaels_CVModel_fast8/Key Outputs/00 Date & Time ==
  u : Inport
  Enable : EnablePort
  DateConversion# : Constant  Value=693960  SampleTime=0.001
  MATLAB Function : MATLAB Function  TreatAsAtomicUnit=on
  Subtract : Sum  Inputs=+-
  DateTime : Outport  SampleTime=0.001
  wires:
  Subtract/1 -> DateTime/1  "DateTime"
  DateConversion#/1 -> Subtract/2
  MATLAB Function/1(D) -> Subtract/1  "DateTime"
  u/1 -> MATLAB Function/1(u)

== system Michaels_CVModel_fast8/Key Outputs/Triggered Subsystem1 ==
  In1 : Inport
  Trigger : TriggerPort  TriggerType=either  FunctionName=Trigger  Variant=on  VariantControl=(inherit)  InitialTriggerSignalState=zero
  Out1 : Outport
  wires:
  In1/1 -> Out1/1

== system Michaels_CVModel_fast8/Key Outputs/Triggered Subsystem2 ==
  In1 : Inport
  Trigger : TriggerPort  TriggerType=either  FunctionName=Trigger  Variant=on  VariantControl=(inherit)  InitialTriggerSignalState=zero
  Out1 : Outport
  wires:
  In1/1 -> Out1/1

== system Michaels_CVModel_fast8/Key Outputs/Triggered Subsystem3 ==
  In1 : Inport
  Trigger : TriggerPort  FunctionName=Trigger  Variant=on  VariantControl=(inherit)  InitialTriggerSignalState=positive
  Out1 : Outport
  wires:
  In1/1 -> Out1/1

== system Michaels_CVModel_fast8/Key Outputs/Triggered Subsystem4 ==
  In1 : Inport
  Enable : EnablePort  StatesWhenEnabling=reset
  Out1 : Outport
  wires:
  In1/1 -> Out1/1

== system Michaels_CVModel_fast8/Key Outputs/Triggered Subsystem5 ==
  In1 : Inport
  Enable : EnablePort  PropagateVarSize=During execution
  Out1 : Outport
  wires:
  In1/1 -> Out1/1

== system Michaels_CVModel_fast8/Key Outputs/Triggered Subsystem6 ==
  In1 : Inport
  Enable : EnablePort  PropagateVarSize=During execution
  Out1 : Outport
  wires:
  In1/1 -> Out1/1
